simulink model "Barrel"  (R2023a)
settings: Solver=VariableStepAuto  StartTime=0.0  StopTime=10.0  RelTol=1e-3
libraries: simulink_extras x1
settings Model: Creator=asd19005  LastModifiedBy=aan18022

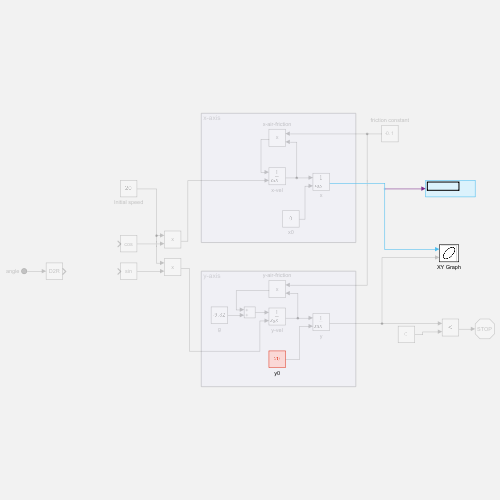
[thumbnail: Simulink's stored preview of the top-level diagram]
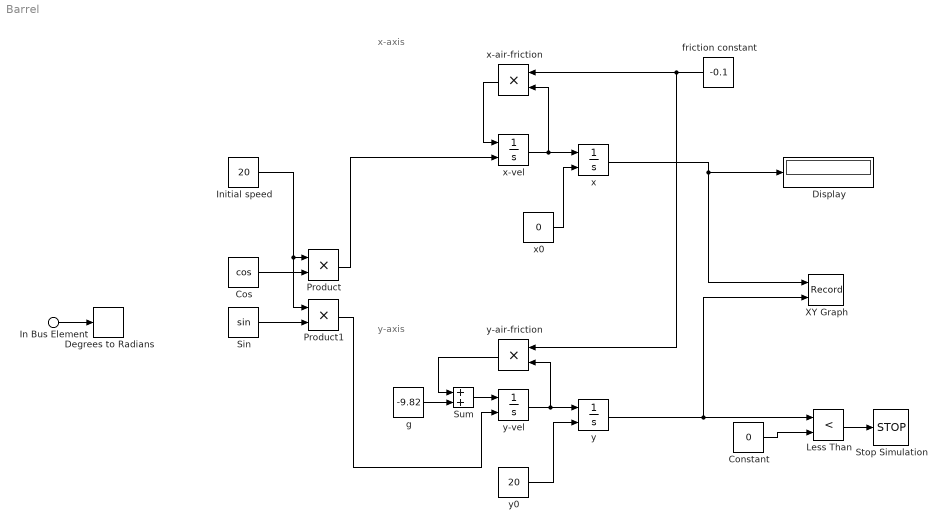
== system Barrel ==
  note: y-axis
  note: x-axis
  In Bus Element : Inport  PortName=angle
  Constant : Constant  Value=0
  Cos : Trigonometry  Operator=cos
  Degrees to Radians : simulink_extras/Transformations/Degrees to Radians
  Display : Display
  Initial speed : Constant  Value=20
  Less Than : RelationalOperator  Operator=<  OutDataTypeStr=boolean  RndMeth=Simplest  InputSameDT=off
  Product : Product
  Product1 : Product
  Sin : Trigonometry
  Stop Simulation : Stop
  Sum : Sum
  XY Graph : Record  FileSettingsInternal="{\"entries\":[{\"content\":{\"excelSettings\":{\"content\":{},\"type\":\"Streamout.ExcelSettings\"}},\"type\":\"Streamout.FileSettingStorage\",\"uuid\":\"fcbac73c-9657-47e5-b741-cd666dd00872\"}],\"packageUris\":[\"http://schema.mathworks.com/mf0/streamout_blocks/R2020a\"],\"version\":\"1.0\"}"  Layout=[1 1]  SignalsInternal="{\"entries\":[{\"content\":{\"signals\":[{\"content\":{\"blockPath\":[\"targetFile/XY Graph\"],\"dimensions\":[1],\"domain\":\"targetFile/XY Graph\",\"lineColor\":\"#77ac30\",\"port\":1,\"signalID\":56,\"signalName\":\"x\"},\"type\":\"RecordBlkView.Signal\",\"uuid\":\"7993c838-46f6-42fe-b134-85c8190fe95e\"},{\"content\":{\"blockPath\":[\"targetFile/XY Graph\"],\"dimensions\":[1],\"domain\":\"targetFile/XY Graph\",\"lineColor\":\"#4dbeee\",\"port\":2,\"signalID\":59,\"signalName\":\"y\"},\"type\":\"RecordBlkView.Signal\",\"uuid\":\"b719affc-30ae-4cf5-9f94-a895b1fc1ad5\"}]},\"type\":\"RecordBlkView.InputSignals\",\"uuid\":\"035ba5e6-d788-4e27-9241-d7c8b68130bb\"}],\"packageUris\":[\"http://schema.mathworks.com/mf0/streamout_blocks/R2020a\"],\"version\":\"1.0\"}"  VisualizationBindings="{\"xyplotplugin\":{\"info\":[{\"series\":[],\"subplotID\":1}]}}"  CompatibilityTag=XY
  friction constant : Constant  Value=-0.1
  g : Constant  Value=-9.82
  x : Integrator  InitialConditionSource=external  InitialCondition=100
  x-air-friction : Product
  x-vel : Integrator  InitialConditionSource=external  InitialCondition=10
  x0 : Constant  Value=0
  y : Integrator  InitialConditionSource=external  InitialCondition=100
  y-air-friction : Product
  y-vel : Integrator  InitialConditionSource=external  InitialCondition=10
  y0 : Constant  Value=20
  wires:
  friction constant/1 -> y-air-friction/1, x-air-friction/1
  x/1 -> Display/1, XY Graph/1
  y-air-friction/1 -> Sum/1
  Less Than/1 -> Stop Simulation/1
  g/1 -> Sum/2
  Product/1 -> x-vel/2
  x-air-friction/1 -> x-vel/1
  Sum/1 -> y-vel/1
  y0/1 -> y/2
  x0/1 -> x/2
  Constant/1 -> Less Than/2
  y-vel/1 -> y-air-friction/2, y/1
  Product1/1 -> y-vel/2
  y/1 -> XY Graph/2, Less Than/1
  x-vel/1 -> x-air-friction/2, x/1
  Sin/1 -> Product1/2
  Cos/1 -> Product/2
  Initial speed/1 -> Product1/1, Product/1
  In Bus Element/1 -> Degrees to Radians/1
